simulink model "pll_sequence_test"  (R2022b)
settings: Solver=VariableStepAuto  StartTime=0.0  StopTime=10.0  RelTol=1e-3  EnableMultiTasking=on
undefined symbols (not defined in the file): DiscIntNeverNeededParam
libraries: powerlib_extras x5, c2802xlib x3, spsFirstOrderFilterLib x3, simulink x1, spsabctodq0Lib x1
settings Model: Creator=menna  LastModifiedBy=menna
settings SolverCC: PositivePriorityOrder=on
settings OptimizationCC: EnhancedBackFolding=on  PassReuseOutputArgsAs=Individual arguments  ZeroExternalMemoryAtStartup=off  ZeroInternalMemoryAtStartup=off  MaxStackSize=64  OptimizeBlockOrder=speed  DifferentSizesBufferReuse=on  OptimizationCustomize=off  EfficientTunableParamExpr=on
settings DebuggingCC: ParameterTunabilityLossMsg=error
settings HardwareCC: ProdBitPerChar=16  ProdBitPerInt=16  ProdBitPerPointer=32  ProdBitPerSizeT=32  ProdBitPerPtrDiffT=32  ProdLargestAtomicInteger=Integer  ProdLargestAtomicFloat=None  ProdWordSize=16  ProdHWDeviceType=Texas Instruments->C2000  HardwareBoardFeatureSet=SoCBlockset
settings ModelReferenceCC: ModelReferenceNumInstancesAllowed=Single
settings SFSimCC: MATLABDynamicMemAlloc=off
settings RTWCC: Description=Embedded Coder  SystemTargetFile=ert.tlc  HardwareBoard=TI Delfino F28379D LaunchPad  TLCOptions=-aInlineSetEventsForThisBaseRateFcn=TLC_FALSE -aSuppressMultiTaskScheduler=TLC_FALSE -aRateBasedStepFcn=1  TemplateMakefile=ert_default_tmf
settings CodeAppCC: ForceParamTrailComments=on  IgnoreCustomStorageClasses=off  OperatorAnnotations=on  SimulinkDataObjDesc=on  SFDataObjDesc=on  InsertBlockDesc=on
settings ERTTargetCC: ExtModeMexFile=TIC2000ExternalModeOpen  ExtModeIntrfLevel=Level2 - Open

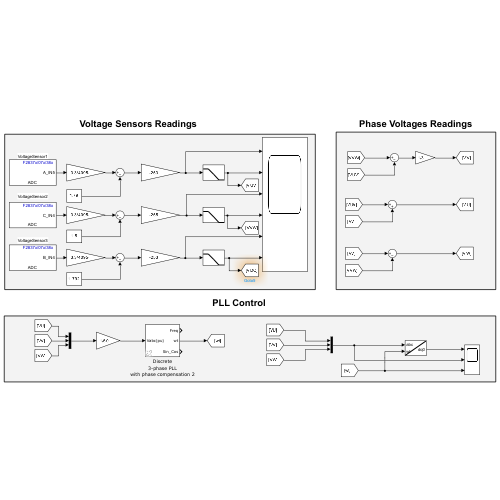
[thumbnail: Simulink's stored preview of the top-level diagram]
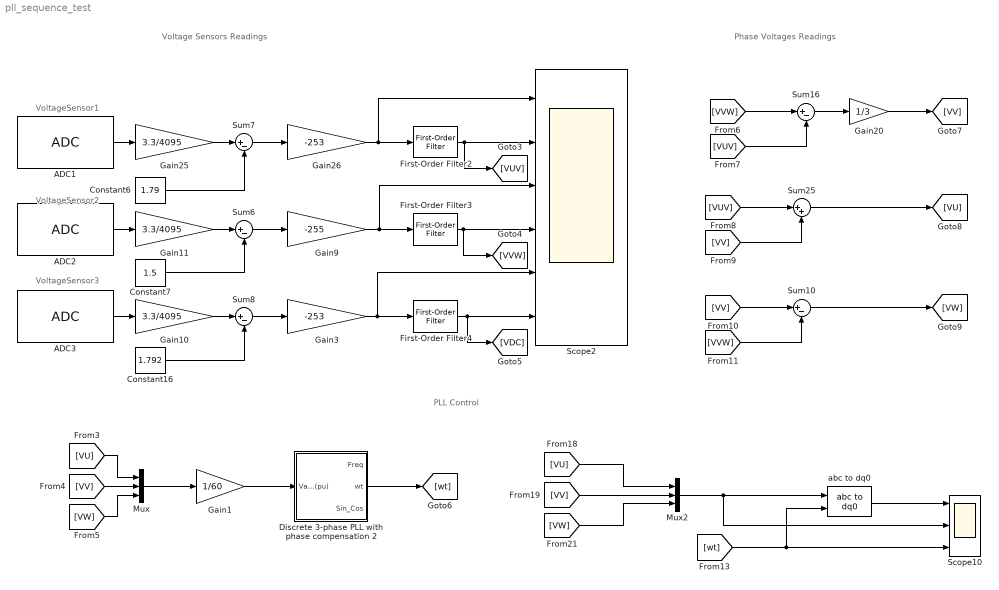
== system pll_sequence_test ==
  note: Phase Voltages Readings
  note: VoltageSensor2
  note: Voltage Sensors Readings
  note: VoltageSensor3
  note: VoltageSensor1
  note: PLL Control
  ADC1 : c2802xlib/ADC  blkParamProc=C2000_Type4  ADCModule=A  samplingMode=Single sample mode  ADCResolution=12-bit (Single-ended input)  useSOC1=SOC0  useSOC2=SOC0_SOC1  SOCAcquisitionWindow=15  SOCTriggerSource=Software  SOCInterruptTrigger=No ADCINT  Ts=1e-4  dType=uint16  postInterrupt=off  interruptSel=ADCINT1  ADCINTContinuous=on  endma=off  chdma=1  conv1=ADCINA0  conv2=ADCINA0 and ADCINB0  conv1_Type4=ADCIN5  conv2_Type4=ADCIN0 and ADCIN1
      settings: LibrarySourceBlock=c2837xDlib/ADC
  ADC2 : c2802xlib/ADC  blkParamProc=C2000_Type4  ADCModule=C  samplingMode=Single sample mode  ADCResolution=12-bit (Single-ended input)  useSOC1=SOC2  useSOC2=SOC0_SOC1  SOCAcquisitionWindow=15  SOCTriggerSource=Software  SOCInterruptTrigger=No ADCINT  Ts=1e-4  dType=uint16  postInterrupt=off  interruptSel=ADCINT1  ADCINTContinuous=on  endma=off  chdma=1  conv1=ADCINA0  conv2=ADCINA0 and ADCINB0  conv1_Type4=ADCIN4  conv2_Type4=ADCIN0 and ADCIN1
      settings: LibrarySourceBlock=c2837xDlib/ADC
  ADC3 : c2802xlib/ADC  blkParamProc=C2000_Type4  ADCModule=B  samplingMode=Single sample mode  ADCResolution=12-bit (Single-ended input)  useSOC1=SOC1  useSOC2=SOC0_SOC1  SOCAcquisitionWindow=15  SOCTriggerSource=Software  SOCInterruptTrigger=No ADCINT  Ts=0.001  dType=uint16  postInterrupt=off  interruptSel=ADCINT1  ADCINTContinuous=on  endma=off  chdma=1  conv1=ADCINA0  conv2=ADCINA0 and ADCINB0  conv1_Type4=ADCIN4  conv2_Type4=ADCIN0 and ADCIN1
      settings: LibrarySourceBlock=c2837xDlib/ADC
  Constant16 : Constant  Value=1.792  SampleTime=-1
  Constant6 : Constant  Value=1.79  SampleTime=-1
  Constant7 : Constant  Value=1.5  SampleTime=-1
  Discrete 3-phase PLL with phase compensation 2 : Subsystem  AncestorBlock=|  DialogController=POWERSYS.PowerSysDialog  mask(Discrete 3-phase PLL){Fmin=45, Par_Init=[0 50], ParK=[ 45 100 0 ], Ts=1e-4, AGC=off}
      | powerlib_extras/Discrete 
      | Control Blocks/Discrete
      | 3-phase PLL
      mask prompts: Fmin "Minimum frequency (Hz):"; Par_Init "Initial inputs:[ Phase(degrees)   Frequency(Hz) ]"; ParK "Regulator gains [ Kp  Ki  Kd ]"; Ts "Sample time:"; AGC "Enable Automatic Gain Control"
      mask help:
      | This Phase Locked Loop (PLL) system can be used  to synchronize on a set of variable frequency, three-phase sinusoidal signals. If the Automatic Gain Control is enabled, the input (phase error) of the PLL regulator is scaled according to the input signals magnitude.
      |
      | For optimal performance, the following settings are recommended:
      |   [ Kp Ki  Kd ] = [ 180  3200  1 ]
      |   "Enable Automatic Gain Control" checked
      |
      | Input 1: Vector containing the normalized three-phase signals [Va Vb Vc]
      | Output 1:  Measured frequency (Hz) = w/(2pi)
      | Output 2:  Ramp w.t varying between  0 and 2*pi,
      |      synchronized on zero crossings of the fundamental (positive-sequence) of phase A.
      | Output 3: Vector [sin(wt) cos(wt)]
      mask init:
      | Kp=ParK(1);
      | Ki=ParK(2);
      | if length(ParK)==2
      |     Kd=0;
      | else
      |     Kd=ParK(3);
      | end    
      | Phase_Init=Par_Init(1);
      | Finit=Par_Init(2);
      | power_initmask();
      settings: OpenFcn=power_openblockproxy();
      settings: LibrarySourceBlock=|
      | powerlib_extras/Discrete
      | Control Blocks/Discrete
      | 3-phase PLL
      mask Help: This block is part of a subset of blocks in the Extras library that does not have documentation associated with it, other than the block mask description.
      mask Display: disp('')
  First-Order Filter2 : spsFirstOrderFilterLib/First-Order Filter  FilterType=Lowpass  Tc=1/250  Ts=1/5000  Initialize=off  Vac_Init=[0, 0, 60]  Vdc_Init=0  PlotResponse=off  FreqRange="[0,  200,  1]"
  First-Order Filter3 : spsFirstOrderFilterLib/First-Order Filter  FilterType=Lowpass  Tc=1/250  Ts=1/5000  Initialize=off  Vac_Init=[0, 0, 60]  Vdc_Init=0  PlotResponse=off  FreqRange="[0,  200,  1]"
  First-Order Filter4 : spsFirstOrderFilterLib/First-Order Filter  FilterType=Lowpass  Tc=1/250  Ts=1/5000  Initialize=off  Vac_Init=[0, 0, 60]  Vdc_Init=0  PlotResponse=off  FreqRange="[0,  200,  1]"
  Gain1 : Gain  Gain=1/60
  Gain10 : Gain  Gain=3.3/4095
  Gain11 : Gain  Gain=3.3/4095
  Gain20 : Gain  Gain=1/3
  Gain25 : Gain  Gain=3.3/4095
  Gain26 : Gain  Gain=-253
  Gain3 : Gain  Gain=-253
  Gain9 : Gain  Gain=-255
  Mux : Mux  Inputs=3
  Mux2 : Mux  Inputs=3
  Scope10 : Scope  NumInputPorts=3
  Scope2 : Scope  NumInputPorts=6
  Sum{6..8,10,16} (5 alike) : Sum  Inputs=|+-
  Sum25 : Sum  Inputs=|++
  abc to dq0 : spsabctodq0Lib/abc to dq0  Alignment=90 degrees behind phase A axis
  wires:
  Sum7/1 -> Gain26/1
  First-Order Filter4/1 -> [VDC], Scope2/6
  Sum10/1 -> [VW]
  [VV] -> Sum25/2
  Gain10/1 -> Sum8/1
  ADC3/1 -> Gain10/1
  [VUV] -> Sum25/1
  [wt] -> abc to dq0/2, Scope10/3
  [VUV] -> Sum16/2
  First-Order Filter3/1 -> Scope2/4, [VVW]
  Constant16/1 -> Sum8/2
  [VW] -> Mux2/3
  ADC2/1 -> Gain11/1
  Mux/1 -> Gain1/1
  Gain3/1 -> First-Order Filter4/1, Scope2/5
  Constant7/1 -> Sum6/2
  Gain25/1 -> Sum7/1
  Mux2/1 -> Scope10/2, abc to dq0/1
  Sum25/1 -> [VU]
  First-Order Filter2/1 -> Scope2/2, [VUV]
  Gain1/1 -> Discrete 3-phase PLL with phase compensation 2/1(Vabc(pu))
  abc to dq0/1 -> Scope10/1
  [VVW] -> Sum16/1
  [VW] -> Mux/3
  [VU] -> Mux2/1
  Gain11/1 -> Sum6/1
  Constant6/1 -> Sum7/2
  [VU] -> Mux/1
  Discrete 3-phase PLL with phase compensation 2/2(wt) -> [wt]
  ADC1/1 -> Gain25/1
  [VVW] -> Sum10/2
  Sum16/1 -> Gain20/1
  Sum6/1 -> Gain9/1
  [VV] -> Mux2/2
  [VV] -> Mux/2
  Gain26/1 -> Scope2/1, First-Order Filter2/1
  Gain20/1 -> [VV]
  Gain9/1 -> Scope2/3, First-Order Filter3/1
  [VV] -> Sum10/1
  Sum8/1 -> Gain3/1

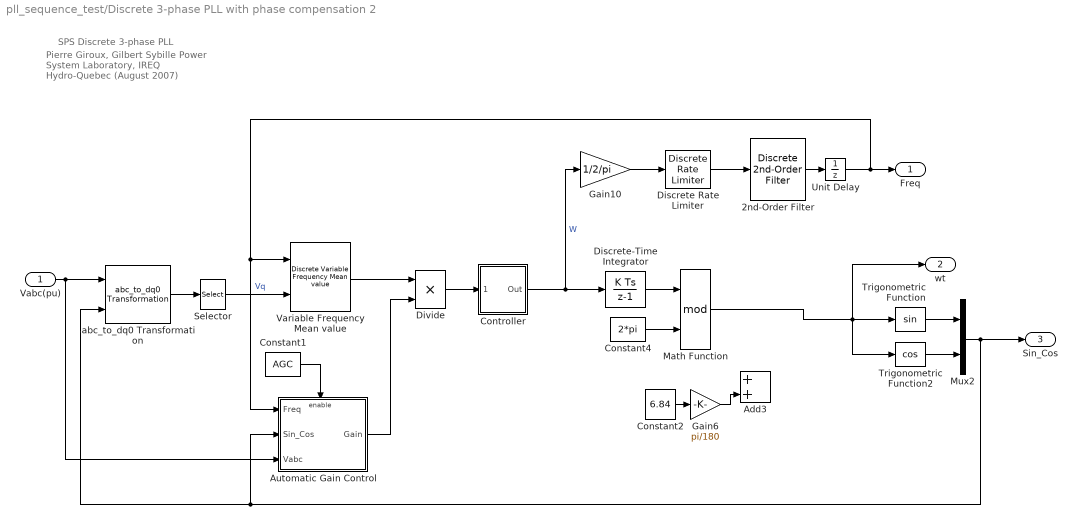
== system pll_sequence_test/Discrete 3-phase PLL with phase compensation 2 ==
  note: SPS Discrete 3-phase PLL
  note: Pierre Giroux, Gilbert Sybille
      | Power System Laboratory, IREQ
      | Hydro-Quebec
      | (August 2007)
  Vabc(pu) : Inport  PortDimensions=3
  2nd-Order Filter : powerlib_extras/Discrete  Control Blocks/Discrete  2nd-Order Filter  FilterType=Lowpass  Fo=25  Zeta=0.707  Ts=Ts  Initialize=on  Vac_Init=[0 0 Finit]  Vdc_Init=Finit  PlotResponse=off  param1=[1 500 0.1]
  Add3 : Sum
  Automatic Gain Control : Subsystem  TreatAsAtomicUnit=on
  Constant1 : Constant  Value=AGC
  Constant2 : Constant  Value=6.84
  Constant4 : Constant  Value=2*pi
  Controller : Subsystem  mask(Discrete PID Controller){Kp=Kp, Ki=Ki, Kd=Kd, Par_Limits=[10000 0], Init=2*pi*Finit, Ts=Ts}
      mask prompts: Kp "Proportional gain (Kp):"; Ki "Integral gain (Ki):"; Kd "Derivative gain (Kd):"; Par_Limits "Output limits: [ Upper   Lower ]"; Init "Output initial value:"; Ts "Sample time:"
      mask help: This block implements a discrete PID controller.
      mask init:
      | UpperLimit=Par_Limits(1);
      | LowerLimit=Par_Limits(2);
      | power_initmask();
      settings: OpenFcn=power_openblockproxy();
      mask Display: disp('PID');
  Discrete Rate Limiter : powerlib_extras/Discrete  Control Blocks/Discrete Rate Limiter  R=12  F=-12  Vinit=Finit  Ts=Ts
  Discrete-Time Integrator : DiscreteIntegrator  InitialCondition=Phase_Init*pi/180  SampleTime=Ts  ICPrevOutput=DiscIntNeverNeededParam  ICPrevScaledInput=DiscIntNeverNeededParam
  Divide : Product
  Gain10 : Gain  Gain=1/2/pi  SaturateOnIntegerOverflow=on  OutDataTypeStr=Inherit: Same as input  ParamDataTypeStr=Inherit: Same as input
  Gain6 : Gain  Gain=pi/180
  Math Function : Math  Operator=mod  SignedPower=on
  Mux2 : Mux  Inputs=2
  Selector : Selector  InputPortWidth=3  IndexOptions=Index vector (dialog)  Indices=2  OutputSizes=1
  Trigonometric Function : Trigonometry
  Trigonometric Function2 : Trigonometry  Operator=cos
  Unit Delay : UnitDelay  InitialCondition=Finit  SampleTime=Ts  HasFrameUpgradeWarning=on
  Variable Frequency Mean value : powerlib_extras/Discrete Measurements/Discrete Variable Frequency Mean value  Finit=Finit  Fmin=Fmin  Vinit=0  Ts=Ts
  abc_to_dq0 Transformation : powerlib_extras/Measurements/abc_to_dq0 Transformation
  Freq : Outport
  wt : Outport  Port=2
  Sin_Cos : Outport  Port=3
  wires:
  Math Function/1 -> Trigonometric Function/1, wt/1, Trigonometric Function2/1
  Constant2/1 -> Gain6/1
  Gain6/1 -> Add3/2
  Constant1/1 -> Automatic Gain Control/Enable
  Divide/1 -> Controller/1(Error)
  Automatic Gain Control/1(Gain) -> Divide/2
  Variable Frequency Mean value/1 -> Divide/1
  Controller/1(Out) -> Gain10/1, Discrete-Time Integrator/1  "W"
  Vabc(pu)/1 -> Automatic Gain Control/3(Vabc), abc_to_dq0 Transformation/1
  abc_to_dq0 Transformation/1 -> Selector/1
  Constant4/1 -> Math Function/2
  Discrete-Time Integrator/1 -> Math Function/1
  Trigonometric Function/1 -> Mux2/1
  Trigonometric Function2/1 -> Mux2/2
  Mux2/1 -> Automatic Gain Control/2(Sin_Cos), abc_to_dq0 Transformation/2, Sin_Cos/1
  Gain10/1 -> Discrete Rate Limiter/1
  Discrete Rate Limiter/1 -> 2nd-Order Filter/1
  Unit Delay/1 -> Automatic Gain Control/1(Freq), Variable Frequency Mean value/1, Freq/1
  2nd-Order Filter/1 -> Unit Delay/1
  Selector/1 -> Variable Frequency Mean value/2  "Vq"

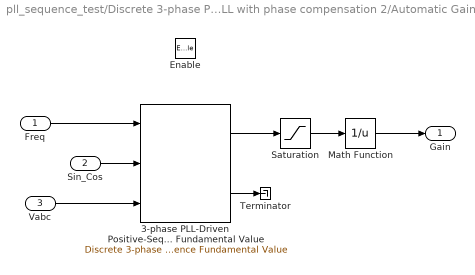
== system pll_sequence_test/Discrete 3-phase PLL with phase compensation 2/Automatic Gain Control ==
  Freq : Inport
  Sin_Cos : Inport  Port=2
  Vabc : Inport  Port=3
  Enable : EnablePort  PropagateVarSize=During execution
  3-phase PLL-Driven Positive-Sequence Fundamental Value : powerlib_extras/Discrete Measurements/Discrete 3-phase PLL-Driven Positive-Sequence Fundamental Value  Finit=Finit  Fmin=Fmin  Par_Init=[1 0]  Ts=Ts
  Math Function : Math  Operator=reciprocal  SignedPower=on
  Saturation : Saturate  UpperLimit=2  LowerLimit=0.01
  Terminator : Terminator
  Gain : Outport  InitialOutput=[1]
  wires:
  Math Function/1 -> Gain/1
  Vabc/1 -> 3-phase PLL-Driven Positive-Sequence Fundamental Value/3
  Sin_Cos/1 -> 3-phase PLL-Driven Positive-Sequence Fundamental Value/2
  Freq/1 -> 3-phase PLL-Driven Positive-Sequence Fundamental Value/1
  3-phase PLL-Driven Positive-Sequence Fundamental Value/1 -> Saturation/1
  Saturation/1 -> Math Function/1
  3-phase PLL-Driven Positive-Sequence Fundamental Value/2 -> Terminator/1

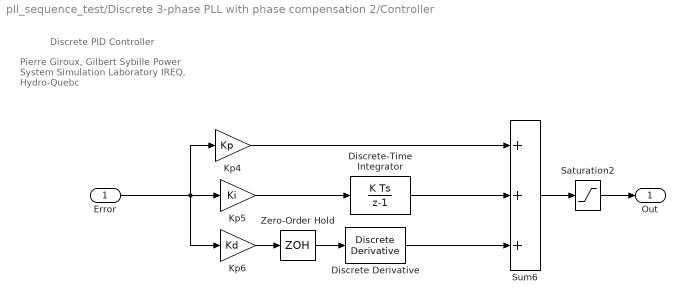
== system pll_sequence_test/Discrete 3-phase PLL with phase compensation 2/Controller ==
  note: Discrete PID Controller
  note: Pierre Giroux, Gilbert Sybille
      | Power System Simulation Laboratory
      | IREQ, Hydro-Quebc
  Error : Inport
  Discrete Derivative : simulink/Discrete/Discrete Derivative  gainval=1.0  ICPrevScaledInput=0.0  OutMin=[]  OutMax=[]  OutDataType=sfix(16)  OutScaling=2^-10  DoSatur=off
  Discrete-Time Integrator : DiscreteIntegrator  InitialCondition=Init  SampleTime=Ts  LimitOutput=on  UpperSaturationLimit=UpperLimit  LowerSaturationLimit=LowerLimit  ICPrevOutput=DiscIntNeverNeededParam  ICPrevScaledInput=DiscIntNeverNeededParam
  Kp4 : Gain  Gain=Kp  SaturateOnIntegerOverflow=on  OutDataTypeStr=Inherit: Same as input  ParamDataTypeStr=Inherit: Same as input
  Kp5 : Gain  Gain=Ki  SaturateOnIntegerOverflow=on  OutDataTypeStr=Inherit: Same as input  ParamDataTypeStr=Inherit: Same as input
  Kp6 : Gain  Gain=Kd  SaturateOnIntegerOverflow=on  OutDataTypeStr=Inherit: Same as input  ParamDataTypeStr=Inherit: Same as input
  Saturation2 : Saturate  UpperLimit=UpperLimit  LowerLimit=LowerLimit
  Sum6 : Sum  Inputs=+++  InputSameDT=on  SaturateOnIntegerOverflow=on  OutDataTypeStr=Inherit: Same as first input
  Zero-Order Hold : ZeroOrderHold  SampleTime=Ts
  Out : Outport  InitialOutput=0
  wires:
  Zero-Order Hold/1 -> Discrete Derivative/1
  Saturation2/1 -> Out/1
  Discrete Derivative/1 -> Sum6/3
  Discrete-Time Integrator/1 -> Sum6/2
  Kp4/1 -> Sum6/1
  Kp6/1 -> Zero-Order Hold/1
  Kp5/1 -> Discrete-Time Integrator/1
  Sum6/1 -> Saturation2/1
  Error/1 -> Kp6/1, Kp5/1, Kp4/1
